simulink model "FourteenBusModel"  (R2021a)
settings: Solver=ode113  StartTime=0.0  StopTime=4  RelTol=1e-3
undefined symbols (not defined in the file): Discrete, linsys1, Time
libraries: spsThreePhaseVIMeasurementLib x47, spsThreePhasePISectionLineLib x20, simulink x13, spsThreePhaseSeriesRLCLoadLib x12, spsThreePhaseTransformerTwoWindingsLib x5, spsPMUPLLBasedPositiveSequenceLib x4, commrandsrc3 x4, ctrlSharedLib x3, spsThreePhaseDynamicLoadLib x3, spsSynchronousMachinepuStandardLib x3, spsThreePhaseParallelRLCLoadLib x3, spsExcitationSystemLib x3
(part 1 of 4)
settings Model: Creator=root  LastModifiedBy=suman
settings SolverCC: AlgebraicLoopSolver=TrustRegion
settings DataIOCC: SaveFormat=Array  SaveOutput=off  SignalLogging=off  DSMLogging=off  SaveTime=off  ReturnWorkspaceOutputs=off
settings DebuggingCC: SFMachineParentedDataDiag=warning  ArithmeticOperatorsInVariantConditions=warning
settings SFSimCC: CustomCodeUndefinedFunction=UseInterfaceOnly

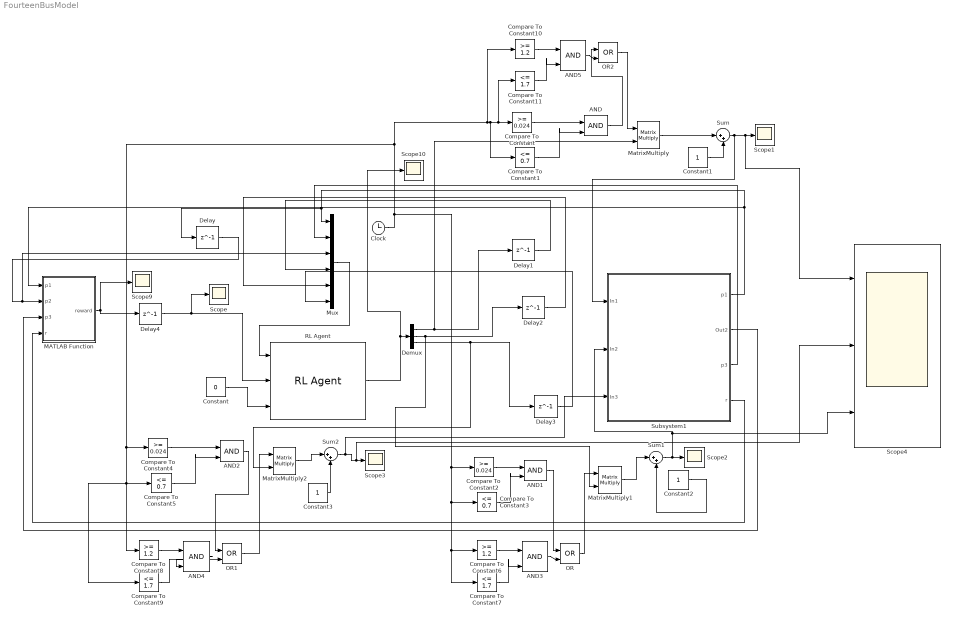
== system FourteenBusModel ==
  AND{,1..5} (6 alike) : Logic  IconShape=distinctive  AllPortsSameDT=off  OutDataTypeStr=boolean
  Clock : Clock
  Compare To Constant : simulink/Logic and Bit Operations/Compare To Constant  relop=>=  const=0.024  OutDataTypeStr=boolean
  Compare To Constant1 : simulink/Logic and Bit Operations/Compare To Constant  relop=<=  const=0.7  OutDataTypeStr=boolean
  Compare To Constant10 : simulink/Logic and Bit Operations/Compare To Constant  relop=>=  const=1.2  OutDataTypeStr=boolean
  Compare To Constant11 : simulink/Logic and Bit Operations/Compare To Constant  relop=<=  const=1.7  OutDataTypeStr=boolean
  Compare To Constant2 : simulink/Logic and Bit Operations/Compare To Constant  relop=>=  const=0.024  OutDataTypeStr=boolean
  Compare To Constant3 : simulink/Logic and Bit Operations/Compare To Constant  relop=<=  const=0.7  OutDataTypeStr=boolean
  Compare To Constant4 : simulink/Logic and Bit Operations/Compare To Constant  relop=>=  const=0.024  OutDataTypeStr=boolean
  Compare To Constant5 : simulink/Logic and Bit Operations/Compare To Constant  relop=<=  const=0.7  OutDataTypeStr=boolean
  Compare To Constant6 : simulink/Logic and Bit Operations/Compare To Constant  relop=>=  const=1.2  OutDataTypeStr=boolean
  Compare To Constant7 : simulink/Logic and Bit Operations/Compare To Constant  relop=<=  const=1.7  OutDataTypeStr=boolean
  Compare To Constant8 : simulink/Logic and Bit Operations/Compare To Constant  relop=>=  const=1.2  OutDataTypeStr=boolean
  Compare To Constant9 : simulink/Logic and Bit Operations/Compare To Constant  relop=<=  const=1.7  OutDataTypeStr=boolean
  Constant : Constant  Value=0
  Constant1 : Constant
  Constant2 : Constant
  Constant3 : Constant
  Delay{,1..4} (5 alike) : Delay  DelayLength=1
  Demux : Demux  Outputs=3
  MATLAB Function : MATLAB Function  TreatAsAtomicUnit=on
  MatrixMultiply : Product  Multiplication=Matrix(*)
  MatrixMultiply1 : Product  Multiplication=Matrix(*)
  MatrixMultiply2 : Product  Multiplication=Matrix(*)
  Mux : Mux  Inputs=6
  OR : Logic  Operator=OR  IconShape=distinctive  AllPortsSameDT=off  OutDataTypeStr=boolean
  OR1 : Logic  Operator=OR  IconShape=distinctive  AllPortsSameDT=off  OutDataTypeStr=boolean
  OR2 : Logic  Operator=OR  IconShape=distinctive  AllPortsSameDT=off  OutDataTypeStr=boolean
  RL Agent : rllib/RL Agent  Agent=agent1  ExternalActionAsInput=off  ProvideCumRwd=off  TreatAsDirectFeedthrough=on
  Scope{,1..3,9..10} (6 alike) : Scope
  Scope4 : Scope  NumInputPorts=3
  Subsystem1 : Subsystem
  Sum : Sum  Inputs=|++
  Sum1 : Sum  Inputs=|++
  Sum2 : Sum  Inputs=|++
  wires:
  MATLAB Function/1(reward) -> Scope9/1, Delay4/1
  Mux/1 -> RL Agent/1
  RL Agent/1 -> Scope10/1, Demux/1
  Delay/1 -> Mux/3, MATLAB Function/2(p2)
  Delay1/1 -> Mux/4
  Delay2/1 -> Mux/5
  Delay3/1 -> Mux/6
  Constant/1 -> RL Agent/3
  Demux/1 -> MatrixMultiply/2, Delay1/1
  Subsystem1/1(p1) -> MATLAB Function/1(p1), Delay/1, Mux/1
  Subsystem1/3(p3) -> Mux/2
  Compare To Constant/1 -> AND/1
  Compare To Constant1/1 -> AND/2
  Demux/2 -> MatrixMultiply1/2, Delay2/1
  Compare To Constant3/1 -> AND1/2
  Compare To Constant2/1 -> AND1/1
  MatrixMultiply1/1 -> Sum1/1
  Demux/3 -> Delay3/1, MatrixMultiply2/2
  Compare To Constant5/1 -> AND2/2
  Clock/1 -> Compare To Constant7/1, Compare To Constant6/1, Compare To Constant3/1, Compare To Constant2/1, Compare To Constant5/1, Compare To Constant9/1, Compare To Constant8/1, Compare To Constant4/1, Compare To Constant10/1, Compare To Constant1/1, Compare To Constant11/1, Compare To Constant/1
  Compare To Constant4/1 -> AND2/1
  MatrixMultiply2/1 -> Sum2/1
  MatrixMultiply/1 -> Sum/1
  Subsystem1/2(Out2) -> MATLAB Function/3(p3)
  Subsystem1/4(r) -> MATLAB Function/4(r)
  Delay4/1 -> Scope/1, RL Agent/2
  Sum/1 -> Subsystem1/1(In1), Scope4/1, Scope1/1
  Constant1/1 -> Sum/2
  Sum1/1 -> Scope4/3, Subsystem1/2(In2), Scope2/1
  Constant2/1 -> Sum1/2
  Sum2/1 -> Subsystem1/3(In3), Scope4/2, Scope3/1
  Constant3/1 -> Sum2/2
  AND1/1 -> OR/1
  Compare To Constant6/1 -> AND3/1
  Compare To Constant7/1 -> AND3/2
  AND3/1 -> OR/2
  OR/1 -> MatrixMultiply1/1
  Compare To Constant9/1 -> AND4/2
  AND4/1 -> OR1/2
  Compare To Constant8/1 -> AND4/1
  AND2/1 -> OR1/1
  OR1/1 -> MatrixMultiply2/1
  Compare To Constant11/1 -> AND5/2
  AND5/1 -> OR2/2
  Compare To Constant10/1 -> AND5/1
  AND/1 -> OR2/1
  OR2/1 -> MatrixMultiply/1
